simulink model "ROB2_schema_Dzvonar"  (R2024b)
settings: Solver=VariableStepAuto  StartTime=0.0  StopTime=20  RelTol=1e-3
undefined symbols (not defined in the file): B1, B2, q1ref, q2ref
libraries: slpidlib x2
settings Model: Creator=imric  LastModifiedBy=imric
settings DebuggingCC: AlgebraicLoopMsg=none

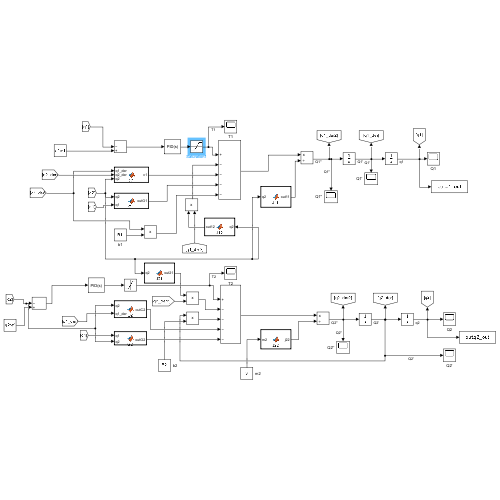
[thumbnail: Simulink's stored preview of the top-level diagram]
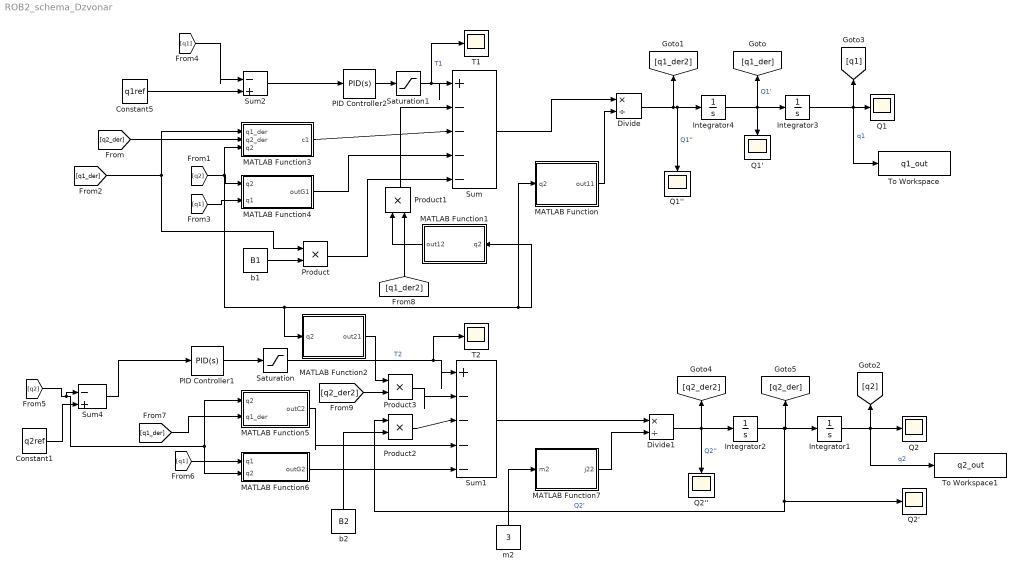
== system ROB2_schema_Dzvonar ==
  Constant1 : Constant  Value=q2ref
  Constant5 : Constant  Value=q1ref
  Divide : Product  Inputs=*/
  Divide1 : Product  Inputs=*/
  Integrator1 : Integrator  InitialCondition=170
  Integrator2 : Integrator
  Integrator3 : Integrator  InitialCondition=170
  Integrator4 : Integrator
  MATLAB Function : MATLAB Function  TreatAsAtomicUnit=on
  MATLAB Function1 : MATLAB Function  TreatAsAtomicUnit=on
  MATLAB Function2 : MATLAB Function  TreatAsAtomicUnit=on
  MATLAB Function3 : MATLAB Function  TreatAsAtomicUnit=on
  MATLAB Function4 : MATLAB Function  TreatAsAtomicUnit=on
  MATLAB Function5 : MATLAB Function  TreatAsAtomicUnit=on
  MATLAB Function6 : MATLAB Function  TreatAsAtomicUnit=on
  MATLAB Function7 : MATLAB Function  TreatAsAtomicUnit=on
  PID Controller1 : slpidlib/PID Controller  Controller=PID  Form=Parallel  TimeDomain=Continuous-time  UseExternalTs=off  SampleTime=-1  IntegratorMethod=Forward Euler  FilterMethod=Forward Euler  ControllerParametersSource=internal  P=275  I=3  UseKiTs=off  D=25  UseExternalDerivativeSource=off  N=100  UseFilter=on  TunerSelectOption=Transfer Function Based (PID Tuner App)  InitialConditionSource=internal  InitialConditionForIntegrator=0  InitialConditionForFilter=0  DifferentiatorICPrevScaledInput=0  ExternalReset=none  TrackingMode=off  Kt=1  LimitOutput=off  SatLimitsSource=internal  UpperSaturationLimit=inf  LowerSaturationLimit=-inf  LinearizeAsGain=on  AntiWindupMode=none  Kb=1  LimitIntegrator=off  UpperIntegratorSaturationLimit=inf  LowerIntegratorSaturationLimit=-inf  POutMin=[]  POutMax=[]  IOutMin=[]  IOutMax=[]  DOutMin=[]  DOutMax=[]  NOutMin=[]  NOutMax=[]  SumOutMin=[]  SumOutMax=[]  SaturationOutMin=[]  SaturationOutMax=[]  PParamMin=[]  PParamMax=[]  IParamMin=[]  IParamMax=[]  DParamMin=[]  DParamMax=[]  NParamMin=[]  NParamMax=[]  KbParamMin=[]  KbParamMax=[]  KtParamMin=[]  KtParamMax=[]  KbOutMin=[]  KbOutMax=[]  KtOutMin=[]  KtOutMax=[]  IntegratorOutMin=[]  IntegratorOutMax=[]  FilterOutMin=[]  FilterOutMax=[]  SumI1OutMin=[]  SumI1OutMax=[]  SumI2OutMin=[]  SumI2OutMax=[]  SumI3OutMin=[]  SumI3OutMax=[]  SumI4OutMin=[]  SumI4OutMax=[]  SumDOutMin=[]  SumDOutMax=[]  DifferentiatorOutMin=[]  DifferentiatorOutMax=[]  FilterDiffOutCoefMin=[]  FilterDiffOutCoefMax=[]  ReciprocalOutMin=[]  ReciprocalOutMax=[]  SumDenOutMin=[]  SumDenOutMax=[]  SumNumOutMin=[]  SumNumOutMax=[]  DivideOutMin=[]  DivideOutMax=[]  UdiffTsProdOutMin=[]  UdiffTsProdOutMax=[]  NTsProdOutMin=[]  NTsProdOutMax=[]  UintegralTsProdOutMin=[]  UintegralTsProdOutMax=[]  UngainTsProdOutMin=[]  UngainTsProdOutMax=[]  ClampingZeroOutDataTypeStr=Inherit: Inherit via back propagation  ClampingZeroOutMin=[]  ClampingZeroOutMax=[]  FilterDenConstantOutDataTypeStr=Inherit: Inherit via back propagation  FilterDenConstantOutMin=[]  FilterDenConstantOutMax=[]  PCopyOutDataTypeStr=Inherit: Inherit via back propagation  PCopyOutMin=[]  PCopyOutMax=[]  NCopyOutDataTypeStr=Inherit: Inherit via back propagation  NCopyOutMin=[]  NCopyOutMax=[]  IntegratorContinuousStateAttributes=''  IntegratorStateMustResolveToSignalObject=off  IntegratorRTWStateStorageClass=Auto  FilterContinuousStateAttributes=''  FilterStateMustResolveToSignalObject=off  FilterRTWStateStorageClass=Auto  ParallelPVariant=InternalParameters  IdealPVariant=Disabled  IVariant=InternalParameters  DVariant=InternalParameters  IntegratorVariant=Continuous  SatVariant=Disabled  AWVariant=Passthrough  PCopyVariant=Disabled  TRVariant=Disabled  FdbkBlocksVariant=Forward  IdealPFdbkVariant=Disabled  SatFdbkVariant=Disabled  DerivativeFilterVariant=ContFilter  NVariant=InternalParameters  NCopyVariant=Disabled  FilterICVariant=InternalICsFilter  IntegratorICVariant=InternalICs  ExternalResetVariant=Disabled  TRSumVariant=Passthrough  SumFdbkVariant=Disabled  SumVariant=Sum_PID  TsampFilterVariant=InternalTs  TsampNgainVariant=Passthrough  TsampIntegralVariant=Disabled_SignalSpec  ExternalSaturationOutDataTypeStr=Inherit: Same as second input  DerivativeSourceVariant=ErrorSignal  PreIntVariant=InternalPreInt
  PID Controller2 : slpidlib/PID Controller  Controller=PID  Form=Parallel  TimeDomain=Continuous-time  UseExternalTs=off  SampleTime=-1  IntegratorMethod=Forward Euler  FilterMethod=Forward Euler  ControllerParametersSource=internal  P=275  I=3  UseKiTs=off  D=125  UseExternalDerivativeSource=off  N=100  UseFilter=on  TunerSelectOption=Transfer Function Based (PID Tuner App)  InitialConditionSource=internal  InitialConditionForIntegrator=0  InitialConditionForFilter=0  DifferentiatorICPrevScaledInput=0  ExternalReset=none  TrackingMode=off  Kt=1  LimitOutput=off  SatLimitsSource=internal  UpperSaturationLimit=inf  LowerSaturationLimit=-inf  LinearizeAsGain=on  AntiWindupMode=none  Kb=1  LimitIntegrator=off  UpperIntegratorSaturationLimit=inf  LowerIntegratorSaturationLimit=-inf  POutMin=[]  POutMax=[]  IOutMin=[]  IOutMax=[]  DOutMin=[]  DOutMax=[]  NOutMin=[]  NOutMax=[]  SumOutMin=[]  SumOutMax=[]  SaturationOutMin=[]  SaturationOutMax=[]  PParamMin=[]  PParamMax=[]  IParamMin=[]  IParamMax=[]  DParamMin=[]  DParamMax=[]  NParamMin=[]  NParamMax=[]  KbParamMin=[]  KbParamMax=[]  KtParamMin=[]  KtParamMax=[]  KbOutMin=[]  KbOutMax=[]  KtOutMin=[]  KtOutMax=[]  IntegratorOutMin=[]  IntegratorOutMax=[]  FilterOutMin=[]  FilterOutMax=[]  SumI1OutMin=[]  SumI1OutMax=[]  SumI2OutMin=[]  SumI2OutMax=[]  SumI3OutMin=[]  SumI3OutMax=[]  SumI4OutMin=[]  SumI4OutMax=[]  SumDOutMin=[]  SumDOutMax=[]  DifferentiatorOutMin=[]  DifferentiatorOutMax=[]  FilterDiffOutCoefMin=[]  FilterDiffOutCoefMax=[]  ReciprocalOutMin=[]  ReciprocalOutMax=[]  SumDenOutMin=[]  SumDenOutMax=[]  SumNumOutMin=[]  SumNumOutMax=[]  DivideOutMin=[]  DivideOutMax=[]  UdiffTsProdOutMin=[]  UdiffTsProdOutMax=[]  NTsProdOutMin=[]  NTsProdOutMax=[]  UintegralTsProdOutMin=[]  UintegralTsProdOutMax=[]  UngainTsProdOutMin=[]  UngainTsProdOutMax=[]  ClampingZeroOutDataTypeStr=Inherit: Inherit via back propagation  ClampingZeroOutMin=[]  ClampingZeroOutMax=[]  FilterDenConstantOutDataTypeStr=Inherit: Inherit via back propagation  FilterDenConstantOutMin=[]  FilterDenConstantOutMax=[]  PCopyOutDataTypeStr=Inherit: Inherit via back propagation  PCopyOutMin=[]  PCopyOutMax=[]  NCopyOutDataTypeStr=Inherit: Inherit via back propagation  NCopyOutMin=[]  NCopyOutMax=[]  IntegratorContinuousStateAttributes=''  IntegratorStateMustResolveToSignalObject=off  IntegratorRTWStateStorageClass=Auto  FilterContinuousStateAttributes=''  FilterStateMustResolveToSignalObject=off  FilterRTWStateStorageClass=Auto  ParallelPVariant=InternalParameters  IdealPVariant=Disabled  IVariant=InternalParameters  DVariant=InternalParameters  IntegratorVariant=Continuous  SatVariant=Disabled  AWVariant=Passthrough  PCopyVariant=Disabled  TRVariant=Disabled  FdbkBlocksVariant=Forward  IdealPFdbkVariant=Disabled  SatFdbkVariant=Disabled  DerivativeFilterVariant=ContFilter  NVariant=InternalParameters  NCopyVariant=Disabled  FilterICVariant=InternalICsFilter  IntegratorICVariant=InternalICs  ExternalResetVariant=Disabled  TRSumVariant=Passthrough  SumFdbkVariant=Disabled  SumVariant=Sum_PID  TsampFilterVariant=InternalTs  TsampNgainVariant=Passthrough  TsampIntegralVariant=Disabled_SignalSpec  ExternalSaturationOutDataTypeStr=Inherit: Same as second input  DerivativeSourceVariant=ErrorSignal  PreIntVariant=InternalPreInt
  Product{,1..3} (4 alike) : Product
  Q1 : Scope
  Q1' : Scope
  Q1'' : Scope
  Q2 : Scope
  Q2' : Scope
  Q2'' : Scope
  Saturation : Saturate  UpperLimit=35  LowerLimit=-35
  Saturation1 : Saturate  UpperLimit=70  LowerLimit=-70
  Sum : Sum  Inputs=|+----
  Sum1 : Sum  Inputs=|+----
  Sum2 : Sum  Inputs=|-+
  Sum4 : Sum  Inputs=|-+
  T1 : Scope
  T2 : Scope
  To Workspace : ToWorkspace  VariableName=q1_out  SampleTime=-1
  To Workspace1 : ToWorkspace  VariableName=q2_out  SampleTime=-1
  b1 : Constant  Value=B1
  b2 : Constant  Value=B2
  m2 : Constant  Value=3
  wires:
  Integrator2/1 -> [q2_der], Integrator1/1, Product2/1, Q2'/1  "Q2'"
  Integrator4/1 -> Q1'/1, [q1_der], Integrator3/1  "Q1'"
  Divide/1 -> Q1''/1, Integrator4/1, [q1_der2]  "Q1''"
  MATLAB Function/1(out11) -> Divide/2
  Sum/1 -> Divide/1
  Product1/1 -> Sum/2
  Divide1/1 -> Q2''/1, [q2_der2], Integrator2/1  "Q2''"
  Sum1/1 -> Divide1/1
  MATLAB Function7/1(j22) -> Divide1/2
  m2/1 -> MATLAB Function7/1(m2)
  b1/1 -> Product/2
  MATLAB Function1/1(out12) -> Product1/1
  MATLAB Function3/1(c1) -> Sum/3
  MATLAB Function4/1(outG1) -> Sum/4
  Integrator3/1 -> To Workspace/1, [q1], Q1/1  "q1"
  Integrator1/1 -> To Workspace1/1, [q2], Q2/1  "q2"
  Constant5/1 -> Sum2/2
  Constant1/1 -> Sum4/2
  MATLAB Function6/1(outG2) -> Sum1/5
  MATLAB Function5/1(outC2) -> Sum1/4
  Product2/1 -> Sum1/3
  b2/1 -> Product2/2
  Product3/1 -> Sum1/2
  MATLAB Function2/1(out21) -> Product3/1
  Product/1 -> Sum/5
  [q1_der] -> MATLAB Function3/1(q1_der), Product/1
  [q2_der] -> MATLAB Function3/2(q2_der)
  [q1] -> MATLAB Function4/2(q1)
  [q2] -> MATLAB Function2/1(q2), MATLAB Function1/1(q2), MATLAB Function/1(q2), MATLAB Function3/3(q2), MATLAB Function4/1(q2)
  [q1] -> Sum2/1
  [q2] -> Sum4/1, MATLAB Function5/1(q2), MATLAB Function6/2(q2)
  [q1] -> MATLAB Function6/1(q1)
  [q1_der] -> MATLAB Function5/2(q1_der)
  [q1_der2] -> Product1/2
  [q2_der2] -> Product3/2
  PID Controller2/1 -> Saturation1/1
  PID Controller1/1 -> Saturation/1
  Saturation/1 -> T2/1, Sum1/1  "T2"
  Saturation1/1 -> T1/1, Sum/1  "T1"
  Sum4/1 -> PID Controller1/1
  Sum2/1 -> PID Controller2/1

== matlab function ROB2_schema_Dzvonar/MATLAB Function ==
  data: out11 output; q2 input
function out11 = J11(q2)
m1 = 3;
m2 = 3; %kg

l1 = 0.25;
l2 = 0.25; %m

g = 9.81; %m*s^-2

j11 = m1*l1^2 + m2 *l1^2 + 2*m2*l1*l2* cos(q2) + m2*l2^2;

out11 = 1/j11;

== matlab function ROB2_schema_Dzvonar/MATLAB Function2 ==
  data: out21 output; q2 input
function out21 = J21(q2)
m2 = 3; %kg

l1 = 0.25;
l2 = 0.25; %m

j21 = m2*l1*l2*cos(q2) + m2*l2^2;

out21 = j21;

== matlab function ROB2_schema_Dzvonar/MATLAB Function3 ==
  data: q1_der input; q2_der input; c1 output; q2 input
function c1 = C1(q1_der,q2_der,q2)

m2 = 3; %kg

l1 = 0.25;
l2 = 0.25; %m

c1 = m2 * l2 * l1 * q2_der * sin(q2)*(2*q1_der+ q2_der);

== matlab function ROB2_schema_Dzvonar/MATLAB Function4 ==
  data: q2 input; outG1 output; q1 input
function outG1 = G1(q2,q1)
m1 = 3;
m2 = 3; %kg

l1 = 0.25;
l2 = 0.25; %m
g =9.81;
outG1 = m1 * g* l1 * cos(q1) + m2 * g * (l1 * cos(q1) + l2 * cos(q1+q2));

== matlab function ROB2_schema_Dzvonar/MATLAB Function5 ==
  data: q2 input; outC2 output; q1_der input
function outC2 = C2(q2,q1_der)

m2 = 3; %kg

l1 = 0.25;
l2 = 0.25; %m

outC2 = m2 * l1 * l2 * q1_der * q1_der * sin(q2);

== matlab function ROB2_schema_Dzvonar/MATLAB Function6 ==
  data: q1 input; outG2 output; q2 input
function outG2 = G2(q1,q2)
m2 = 3; %kg

l2 = 0.25; %m
g = 9.81;

outG2 = m2 * g * l2 * cos(q1+q2);

== matlab function ROB2_schema_Dzvonar/MATLAB Function7 ==
  data: j22 output; m2 input
function j22 = J22(m2)
l2 = 0.25; %m

j22 = m2*l2^2;

== matlab function ROB2_schema_Dzvonar/MATLAB Function1 ==
  data: out12 output; q2 input
function out12 = J12(q2)
m2 = 3; %kg

l1 = 0.25;
l2 = 0.25; %m

j12 = m2*l1*l2*cos(q2) + m2*l2^2;

out12 = j12;
